simulink model "Test_GPS"  (R2024a)
settings: Solver=VariableStepAuto  StartTime=0.0  StopTime=10.0  RelTol=1e-3
libraries: sensorgpslib x1
settings Model: Creator=gerar  LastModifiedBy=gerar

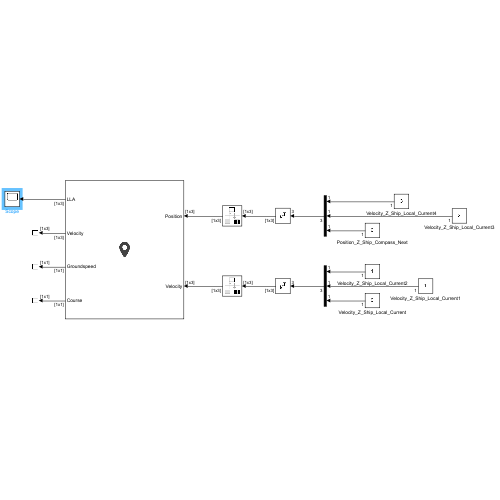
[thumbnail: Simulink's stored preview of the top-level diagram]
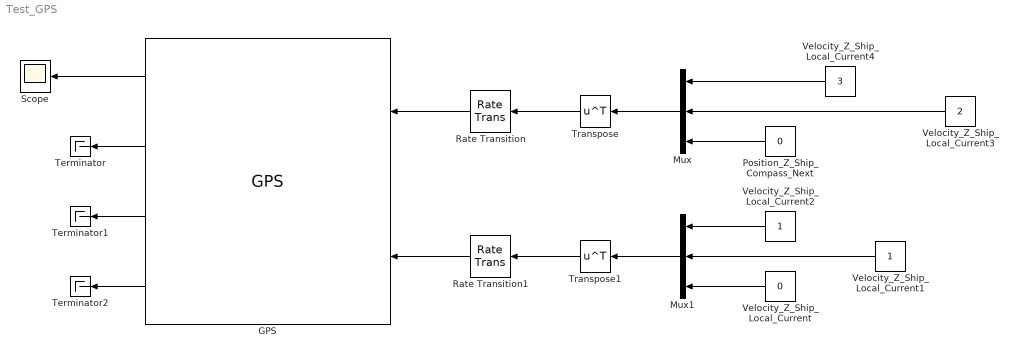
== system Test_GPS ==
  GPS : sensorgpslib/GPS  DispRefFrame=ENU  PositionInputFormat=Local  ReferenceLocation=[43.059023, 3.002915 ,0]  HorizontalPositionAccuracy=1.6  VerticalPositionAccuracy=3  VelocityAccuracy=0.1  DecayFactor=0.999  SeedDouble=67  SimulateUsing=Interpreted execution
  Mux : Mux  Inputs=3
  Mux1 : Mux  Inputs=3
  Position_Z_Ship_Compass_Next : Constant  Value=0
  Rate Transition : RateTransition  OutPortSampleTime=0.01
  Rate Transition1 : RateTransition  OutPortSampleTime=0.01
  Scope : Scope
  Terminator : Terminator
  Terminator1 : Terminator
  Terminator2 : Terminator
  Transpose : Math  Operator=transpose
  Transpose1 : Math  Operator=transpose
  Velocity_Z_Ship_Local_Current : Constant  Value=0
  Velocity_Z_Ship_Local_Current1 : Constant
  Velocity_Z_Ship_Local_Current2 : Constant
  Velocity_Z_Ship_Local_Current3 : Constant  Value=2
  Velocity_Z_Ship_Local_Current4 : Constant  Value=3
  wires:
  GPS/2 -> Terminator/1
  GPS/1 -> Scope/1
  GPS/4 -> Terminator2/1
  GPS/3 -> Terminator1/1
  Mux/1 -> Transpose/1
  Velocity_Z_Ship_Local_Current1/1 -> Mux1/2
  Transpose1/1 -> Rate Transition1/1
  Transpose/1 -> Rate Transition/1
  Position_Z_Ship_Compass_Next/1 -> Mux/3
  Velocity_Z_Ship_Local_Current4/1 -> Mux/1
  Rate Transition/1 -> GPS/1
  Mux1/1 -> Transpose1/1
  Velocity_Z_Ship_Local_Current/1 -> Mux1/3
  Velocity_Z_Ship_Local_Current2/1 -> Mux1/1
  Rate Transition1/1 -> GPS/2
  Velocity_Z_Ship_Local_Current3/1 -> Mux/2
